simulink model "APLRL2D_avoidance_version"  (R2020a)
settings: Solver=ode23t  StartTime=0.0  StopTime=Tf  RelTol=1e-2  EnableMultiTasking=on
PreLoadFcn:
  | robotParametersRL
undefined symbols (not defined in the file or in its folder): Angular, Linear, Pose
libraries: robotlib x12, simulink x6, sharedtransform x1, rllib x1
(part 2 of 2)

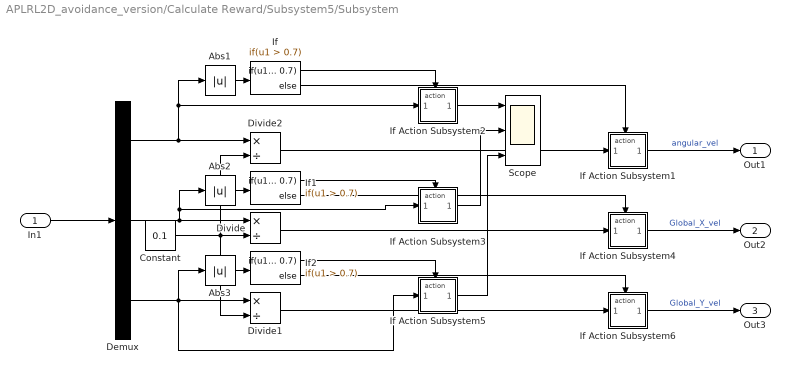
== system APLRL2D_avoidance_version/Calculate Reward/Subsystem5/Subsystem ==
  In1 : Inport
  Abs1 : Abs
  Abs2 : Abs
  Abs3 : Abs
  Constant : Constant  Value=0.1
  Demux : Demux  Outputs=3
  Divide : Product  Inputs=*/
  Divide1 : Product  Inputs=*/
  Divide2 : Product  Inputs=*/
  If : If  IfExpression=u1 > 0.7
  If Action Subsystem1 : Subsystem  TreatAsAtomicUnit=on
  If Action Subsystem2 : Subsystem  TreatAsAtomicUnit=on
  If Action Subsystem3 : Subsystem  TreatAsAtomicUnit=on
  If Action Subsystem4 : Subsystem  TreatAsAtomicUnit=on
  If Action Subsystem5 : Subsystem  TreatAsAtomicUnit=on
  If Action Subsystem6 : Subsystem  TreatAsAtomicUnit=on
  If1 : If  IfExpression=u1 > 0.7
  If2 : If  IfExpression=u1 > 0.7
  Scope : Scope  NumInputPorts=3
  Out1 : Outport
  Out2 : Outport  Port=2
  Out3 : Outport  Port=3
  wires:
  In1/1 -> Demux/1
  Demux/3 -> If Action Subsystem5/1(In1), Abs3/1, Divide1/1
  Divide1/1 -> If Action Subsystem6/1(In1)
  If Action Subsystem3/1(Out1) -> Scope/2
  Divide2/1 -> If Action Subsystem1/1(In1)
  If Action Subsystem5/1(Out1) -> Scope/3
  Abs1/1 -> If/1
  Abs3/1 -> If2/1
  Constant/1 -> Divide1/2, Divide2/2, Divide/2
  Abs2/1 -> If1/1
  Demux/2 -> If Action Subsystem3/1(In1), Abs2/1, Divide/1
  Divide/1 -> If Action Subsystem4/1(In1)
  If Action Subsystem2/1(Out1) -> Scope/1
  Demux/1 -> If Action Subsystem2/1(In1), Abs1/1, Divide2/1
  If Action Subsystem1/1(Out1) -> Out1/1  "angular_vel"
  If Action Subsystem4/1(Out1) -> Out2/1  "Global_X_vel"
  If Action Subsystem6/1(Out1) -> Out3/1  "Global_Y_vel"
  If2/1 -> If Action Subsystem5/Action
  If1/1 -> If Action Subsystem3/Action
  If/1 -> If Action Subsystem2/Action
  If/2 -> If Action Subsystem1/Action
  If1/2 -> If Action Subsystem4/Action
  If2/2 -> If Action Subsystem6/Action

== system APLRL2D_avoidance_version/Check if Done/If Action Subsystem9/Subsystem4 ==
  In1 : Inport
  Data Type Conversion2 : DataTypeConversion  OutDataTypeStr=uint16
  Gain : Gain  Gain=10
  If : If
  If Action Subsystem : Subsystem  TreatAsAtomicUnit=on
  If Action Subsystem1 : Subsystem  TreatAsAtomicUnit=on
  Merge : Merge
  Unit Delay : UnitDelay  SampleTime=-1  HasFrameUpgradeWarning=on
  Out1 : Outport
  wires:
  In1/1 -> Gain/1
  If/1 -> If Action Subsystem/Action
  If/2 -> If Action Subsystem1/Action
  Unit Delay/1 -> If Action Subsystem1/1(In1)
  If Action Subsystem1/1(Out1) -> Merge/2
  If Action Subsystem/1(Out1) -> Merge/1
  Merge/1 -> Out1/1
  Gain/1 -> Data Type Conversion2/1
  Data Type Conversion2/1 -> Unit Delay/1, If Action Subsystem/1(In1), If/1

== system APLRL2D_avoidance_version/Check if Done/Subsystem/Read Model_name ==
  msg : Inport
  Enable : EnablePort
  string : Outport
  wires:
  msg/1 -> string/1

== system APLRL2D_avoidance_version/Calculate Observation/If Action Subsystem1/Subsystem5/If Action Subsystem ==
  In1 : Inport
  Action Port : ActionPort  ActionPortLabel=if(u1 > 0)
  Out1 : Outport
  wires:
  In1/1 -> Out1/1

== system APLRL2D_avoidance_version/Calculate Observation/If Action Subsystem1/Subsystem5/If Action Subsystem1 ==
  In1 : Inport
  Action Port : ActionPort  ActionPortLabel=else
  Out1 : Outport
  wires:
  In1/1 -> Out1/1

== system APLRL2D_avoidance_version/Calculate Observation/If Action Subsystem2/Subsystem4/If Action Subsystem ==
  In1 : Inport
  Action Port : ActionPort  ActionPortLabel=if(u1 > 0)
  Out1 : Outport
  wires:
  In1/1 -> Out1/1

== system APLRL2D_avoidance_version/Calculate Observation/If Action Subsystem2/Subsystem4/If Action Subsystem1 ==
  In1 : Inport
  Action Port : ActionPort  ActionPortLabel=else
  Out1 : Outport
  wires:
  In1/1 -> Out1/1

== system APLRL2D_avoidance_version/Calculate Reward/If Action Subsystem2/Subsystem4/If Action Subsystem ==
  In1 : Inport
  Action Port : ActionPort  ActionPortLabel=if(u1 > 0)
  Out1 : Outport
  wires:
  In1/1 -> Out1/1

== system APLRL2D_avoidance_version/Calculate Reward/If Action Subsystem2/Subsystem4/If Action Subsystem1 ==
  In1 : Inport
  Action Port : ActionPort  ActionPortLabel=else
  Out1 : Outport
  wires:
  In1/1 -> Out1/1

== system APLRL2D_avoidance_version/Calculate Reward/Subsystem/If Action Subsystem2/If Action Subsystem ==
  In1 : Inport
  Action Port : ActionPort  ActionPortLabel=else
  Out1 : Outport
  wires:
  In1/1 -> Out1/1

== system APLRL2D_avoidance_version/Calculate Reward/Subsystem/If Action Subsystem2/If Action Subsystem1 ==
  In1 : Inport
  Action Port : ActionPort  ActionPortLabel=if(u1 > 0)
  Gain : Gain  Gain=-1
  Out1 : Outport
  wires:
  In1/1 -> Gain/1
  Gain/1 -> Out1/1

== system APLRL2D_avoidance_version/Calculate Reward/Subsystem/If Action Subsystem2/If Action Subsystem2 ==
  In1 : Inport
  Action Port : ActionPort  ActionPortLabel=else
  Out1 : Outport
  wires:
  In1/1 -> Out1/1

== system APLRL2D_avoidance_version/Calculate Reward/Subsystem/If Action Subsystem2/If Action Subsystem3 ==
  In1 : Inport
  Action Port : ActionPort  ActionPortLabel=if(u1 > 2.828)
  Gain : Gain  Gain=-1
  Out1 : Outport
  wires:
  In1/1 -> Gain/1
  Gain/1 -> Out1/1

== system APLRL2D_avoidance_version/Calculate Reward/Subsystem/If Action Subsystem3/If Action Subsystem ==
  In1 : Inport
  Action Port : ActionPort  ActionPortLabel=if(u1 > 0)
  Out1 : Outport
  wires:
  In1/1 -> Out1/1

== system APLRL2D_avoidance_version/Calculate Reward/Subsystem/If Action Subsystem3/If Action Subsystem1 ==
  In1 : Inport
  Action Port : ActionPort  ActionPortLabel=else
  Gain : Gain  Gain=-1
  Out1 : Outport
  wires:
  Gain/1 -> Out1/1
  In1/1 -> Gain/1

== system APLRL2D_avoidance_version/Calculate Reward/Subsystem/If Action Subsystem3/Subsystem ==
  In1 : Inport
  Gain2 : Gain  Gain=10
  Math Function : Math  SaturateOnIntegerOverflow=on
  Math Function2 : Math  Operator=square  SaturateOnIntegerOverflow=on
  Out1 : Outport
  wires:
  Math Function2/1 -> Gain2/1
  Gain2/1 -> Math Function/1
  In1/1 -> Math Function2/1
  Math Function/1 -> Out1/1

== system APLRL2D_avoidance_version/Calculate Reward/Subsystem5/Subsystem/If Action Subsystem1 ==
  In1 : Inport
  Action Port : ActionPort  ActionPortLabel=else
  Out1 : Outport
  wires:
  In1/1 -> Out1/1

== system APLRL2D_avoidance_version/Calculate Reward/Subsystem5/Subsystem/If Action Subsystem2 ==
  In1 : Inport
  Action Port : ActionPort  ActionPortLabel=if(u1 > 0.7)
  Out1 : Outport
  wires:
  In1/1 -> Out1/1

== system APLRL2D_avoidance_version/Calculate Reward/Subsystem5/Subsystem/If Action Subsystem3 ==
  In1 : Inport
  Action Port : ActionPort  ActionPortLabel=if(u1 > 0.7)
  Out1 : Outport
  wires:
  In1/1 -> Out1/1

== system APLRL2D_avoidance_version/Calculate Reward/Subsystem5/Subsystem/If Action Subsystem4 ==
  In1 : Inport
  Action Port : ActionPort  ActionPortLabel=else
  Out1 : Outport
  wires:
  In1/1 -> Out1/1

== system APLRL2D_avoidance_version/Calculate Reward/Subsystem5/Subsystem/If Action Subsystem5 ==
  In1 : Inport
  Action Port : ActionPort  ActionPortLabel=if(u1 > 0.7)
  Out1 : Outport
  wires:
  In1/1 -> Out1/1

== system APLRL2D_avoidance_version/Calculate Reward/Subsystem5/Subsystem/If Action Subsystem6 ==
  In1 : Inport
  Action Port : ActionPort  ActionPortLabel=else
  Out1 : Outport
  wires:
  In1/1 -> Out1/1

== system APLRL2D_avoidance_version/Check if Done/If Action Subsystem9/Subsystem4/If Action Subsystem ==
  In1 : Inport
  Action Port : ActionPort  ActionPortLabel=if(u1 > 0)
  Out1 : Outport
  wires:
  In1/1 -> Out1/1

== system APLRL2D_avoidance_version/Check if Done/If Action Subsystem9/Subsystem4/If Action Subsystem1 ==
  In1 : Inport
  Action Port : ActionPort  ActionPortLabel=else
  Out1 : Outport
  wires:
  In1/1 -> Out1/1
